simulink model "slrt_ex_pmsm_original_2022b"  (R2022b)
settings: Solver=FixedStepDiscrete  StartTime=0.0  StopTime=0.25  RelTol=1e-3  EnableMultiTasking=on
PreLoadFcn:
  | Ts = 1e-4;
  | Tcpu = 50e-6; %Controller sample time
  | 
  | % PMSM parameters
  | PM = 0.03; % Permanent magnet flux linkage
  | Ld = 2e-4;  % d-axis inductance
  | Lq = 2e-4;  % q-axis inductance
  | L0 = 2e-4;  % 0-axis inductance
  | Rs = 0.013; % Stator resistance
  | N = 6; % Number of pole pairs
  | J = 0.2; % Moment of inertia
  | 
  | % encoder parameters
  | numSlits = 2000; % number of slits
  | pulseSigOffset = 0; % index pulse signal offset
  | shaftInitPos = 0; % motor shaft initial position
  | 
  | % DAC parameters
  | gain = 0.1;
  | bias = 0;
  | 
  | % circuit parameters
  | Vdc = 48;
  | 
  | % real-time parameters
  | ts_FPGA_clk = 5e-9;
  | ts_FPGA_mdl = 1e-6;
  | 
  | % Real-time processor or embedded controller
  | RTorTTL = 1; % 1: Real-time processor,    0: embedded controller
  | 
  | % sample times
  | f_base = 200e6;
  | PWM_frequency = 20e3;
  | ts_FPGA_clk = 1/f_base;
  | ts_FPGA_mdl =1e-6;
libraries: HDL_Motor_Lib x3, hdlsllib x3, SCA_HDL_CoreMath_Lib x1, simulink x1
settings Model: Creator=The MathWorks, Inc.  LastModifiedBy=mathieu.lu-dac
settings OptimizationCC: BlockReduction=off  ConditionallyExecuteInputs=off  DefaultParameterBehavior=Inlined
settings DebuggingCC: AlgebraicLoopMsg=error  SingleTaskRateTransMsg=error  ParameterPrecisionLossMsg=none
settings HardwareCC: ProdBitPerPointer=32  ProdBitPerSizeT=32  ProdBitPerPtrDiffT=32  ProdLargestAtomicFloat=None  ProdIntDivRoundTo=Undefined  ProdEndianess=Unspecified  ProdWordSize=32  ProdHWDeviceType=ASIC/FPGA->ASIC/FPGA  TargetBitPerPointer=64  TargetBitPerSizeT=64  TargetBitPerPtrDiffT=64  TargetLongLongMode=on  TargetIntDivRoundTo=Zero  TargetEndianess=LittleEndian  TargetWordSize=64  TargetHWDeviceType=Custom Processor->MATLAB Host Computer  ProdEqTarget=off
settings ModelReferenceCC: EnableRefExpFcnMdlSchedulingChecks=on
settings RTWCC: DLArmComputeVersion=19.05

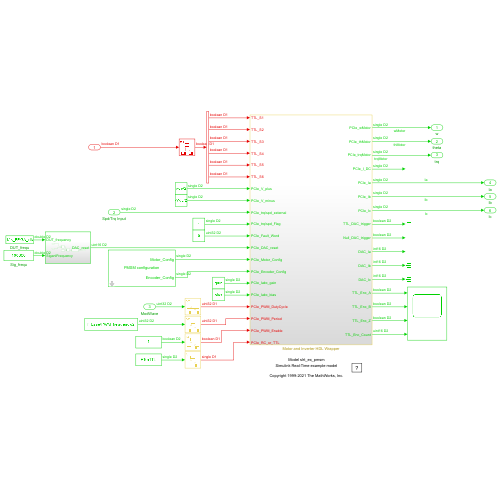
[thumbnail: Simulink's stored preview of the top-level diagram]
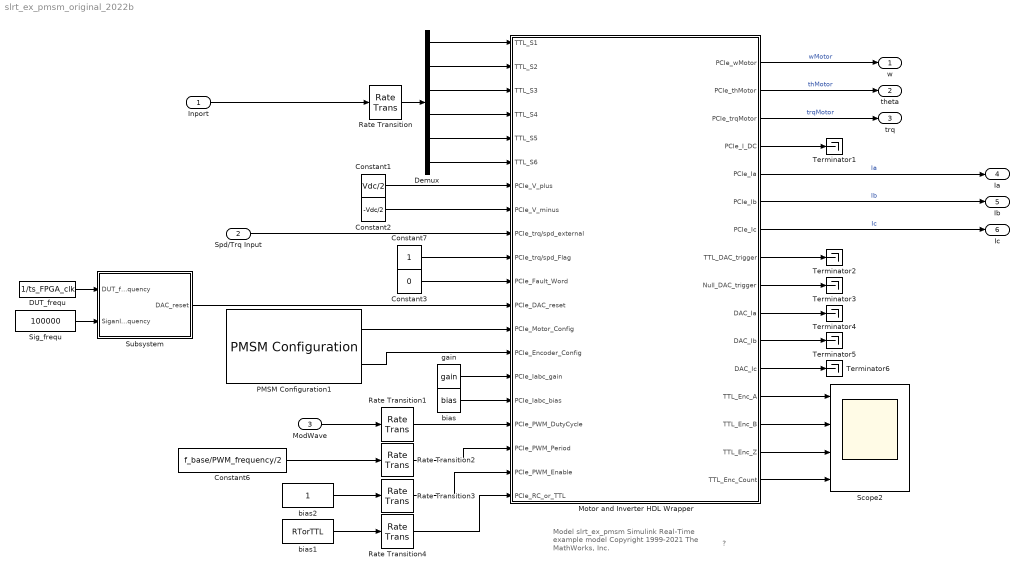
== system slrt_ex_pmsm_original_2022b ==
  note: Model slrt_ex_pmsm
      | Simulink Real-Time example model
      |
      | Copyright 1999-2021 The MathWorks, Inc.
  note: ?
  Inport : Inport  OutDataTypeStr=boolean  PortDimensions=[1 6]
  Spd/Trq Input : Inport  Port=2  OutDataTypeStr=single
  ModWave : Inport  Port=3  OutDataTypeStr=uint32  PortDimensions=[1 3]  SampleTime=ts_FPGA_mdl
  Constant1 : Constant  Value=Vdc/2  OutDataTypeStr=single  SampleTime=ts_FPGA_mdl
  Constant2 : Constant  Value=-Vdc/2  OutDataTypeStr=single  SampleTime=ts_FPGA_mdl
  Constant3 : Constant  Value=0  OutDataTypeStr=uint32  SampleTime=ts_FPGA_mdl
  Constant6 : Constant  Value=f_base/PWM_frequency/2  OutDataTypeStr=uint32  SampleTime=ts_FPGA_mdl
  Constant7 : Constant  OutDataTypeStr=single  SampleTime=ts_FPGA_mdl
  DUT_frequ : Constant  Value=1/ts_FPGA_clk  SampleTime=ts_FPGA_mdl
  Demux : Demux  Outputs=6
  Motor and Inverter HDL Wrapper : Subsystem
  PMSM Configuration1 : HDL_Motor_Lib/PMSM Configuration  Ts=ts_FPGA_mdl  NPP=N  Lambda_pm=PM  Ld=Ld  Lq=Lq  Rs=Rs  J=J  numSlits=numSlits  shaftRotateDir=clockwise (CW)  shaftRotateDirIdx=1  zOffset=pulseSigOffset  shaftInitialPos=shaftInitPos  zGateMode=pulse width = 180 el when channel A is high  zGateModeIdx=1
  Rate Transition{,1..4} (5 alike) : RateTransition  OutPortSampleTime=ts_FPGA_clk
  Scope2 : Scope  NumInputPorts=4
  Sig_frequ : Constant  Value=100000  VectorParams1D=off  SampleTime=ts_FPGA_mdl
  Subsystem : Subsystem
  Terminator{1..6} (6 alike) : Terminator
  bias : Constant  Value=bias  OutDataTypeStr=single  SampleTime=ts_FPGA_mdl
  bias1 : Constant  Value=RTorTTL  OutDataTypeStr=single  SampleTime=ts_FPGA_mdl
  bias2 : Constant  OutDataTypeStr=boolean  SampleTime=ts_FPGA_mdl
  gain : Constant  Value=gain  OutDataTypeStr=single  SampleTime=ts_FPGA_mdl
  w : Outport
  theta : Outport  Port=2
  trq : Outport  Port=3
  Ia : Outport  Port=4
  Ib : Outport  Port=5
  Ic : Outport  Port=6
  wires:
  Rate Transition/1 -> Demux/1
  Demux/1 -> Motor and Inverter HDL Wrapper/1(TTL_S1)
  Demux/2 -> Motor and Inverter HDL Wrapper/2(TTL_S2)
  Demux/3 -> Motor and Inverter HDL Wrapper/3(TTL_S3)
  Demux/4 -> Motor and Inverter HDL Wrapper/4(TTL_S4)
  Demux/5 -> Motor and Inverter HDL Wrapper/5(TTL_S5)
  Demux/6 -> Motor and Inverter HDL Wrapper/6(TTL_S6)
  Constant1/1 -> Motor and Inverter HDL Wrapper/7(PCIe_V_plus)
  Constant2/1 -> Motor and Inverter HDL Wrapper/8(PCIe_V_minus)
  Spd/Trq Input/1 -> Motor and Inverter HDL Wrapper/9(PCIe_trq/spd_external)
  Constant7/1 -> Motor and Inverter HDL Wrapper/10(PCIe_trq/spd_Flag)
  Constant3/1 -> Motor and Inverter HDL Wrapper/11(PCIe_Fault_Word)
  Subsystem/1(DAC_reset) -> Motor and Inverter HDL Wrapper/12(PCIe_DAC_reset)
  Motor and Inverter HDL Wrapper/4(PCIe_I_DC) -> Terminator1/1
  Motor and Inverter HDL Wrapper/8(TTL_DAC_trigger) -> Terminator2/1
  Motor and Inverter HDL Wrapper/9(Null_DAC_trigger) -> Terminator3/1
  Motor and Inverter HDL Wrapper/10(DAC_Ia) -> Terminator4/1
  Motor and Inverter HDL Wrapper/11(DAC_Ib) -> Terminator5/1
  Motor and Inverter HDL Wrapper/12(DAC_Ic) -> Terminator6/1
  Motor and Inverter HDL Wrapper/13(TTL_Enc_A) -> Scope2/1
  Motor and Inverter HDL Wrapper/14(TTL_Enc_B) -> Scope2/2
  Motor and Inverter HDL Wrapper/15(TTL_Enc_Z) -> Scope2/3
  Motor and Inverter HDL Wrapper/16(TTL_Enc_Count) -> Scope2/4
  Inport/1 -> Rate Transition/1
  bias/1 -> Motor and Inverter HDL Wrapper/16(PCIe_Iabc_bias)
  gain/1 -> Motor and Inverter HDL Wrapper/15(PCIe_Iabc_gain)
  Motor and Inverter HDL Wrapper/1(PCIe_wMotor) -> w/1  "wMotor"
  Motor and Inverter HDL Wrapper/2(PCIe_thMotor) -> theta/1  "thMotor"
  Motor and Inverter HDL Wrapper/5(PCIe_Ia) -> Ia/1  "Ia"
  Motor and Inverter HDL Wrapper/6(PCIe_Ib) -> Ib/1  "Ib"
  Motor and Inverter HDL Wrapper/7(PCIe_Ic) -> Ic/1  "Ic"
  DUT_frequ/1 -> Subsystem/1(DUT_frequency)
  Sig_frequ/1 -> Subsystem/2(SiganlFrequency)
  Motor and Inverter HDL Wrapper/3(PCIe_trqMotor) -> trq/1  "trqMotor"
  Constant6/1 -> Rate Transition2/1
  Rate Transition1/1 -> Motor and Inverter HDL Wrapper/17(PCIe_PWM_DutyCycle)
  Rate Transition2/1 -> Motor and Inverter HDL Wrapper/18(PCIe_PWM_Period)
  bias2/1 -> Rate Transition3/1
  Rate Transition3/1 -> Motor and Inverter HDL Wrapper/19(PCIe_PWM_Enable)
  bias1/1 -> Rate Transition4/1
  Rate Transition4/1 -> Motor and Inverter HDL Wrapper/20(PCIe_RC_or_TTL)
  PMSM Configuration1/1 -> Motor and Inverter HDL Wrapper/13(PCIe_Motor_Config)
  PMSM Configuration1/2 -> Motor and Inverter HDL Wrapper/14(PCIe_Encoder_Config)
  ModWave/1 -> Rate Transition1/1

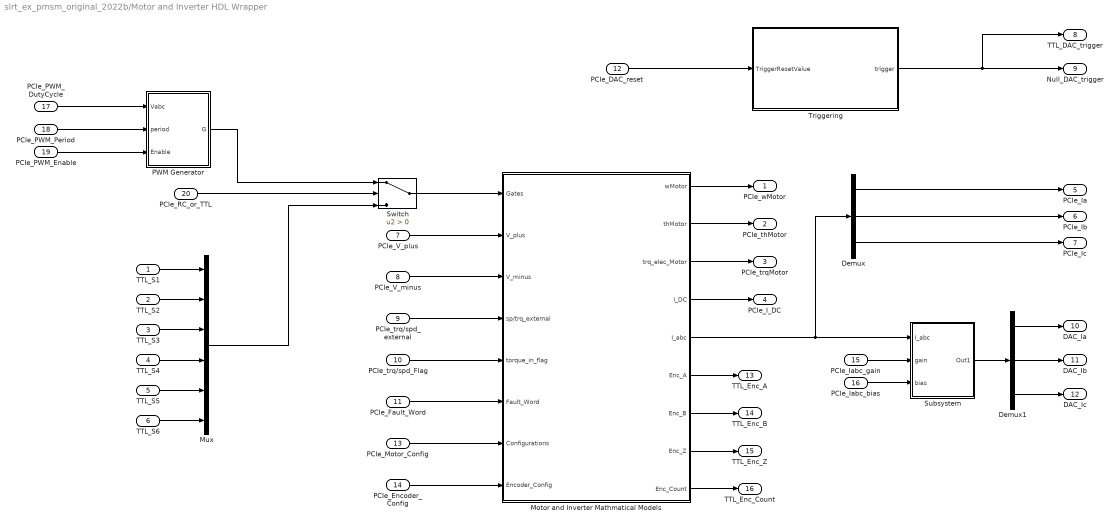
== system slrt_ex_pmsm_original_2022b/Motor and Inverter HDL Wrapper ==
  TTL_S1 : Inport
  TTL_S2 : Inport  Port=2
  TTL_S3 : Inport  Port=3
  TTL_S4 : Inport  Port=4
  TTL_S5 : Inport  Port=5
  TTL_S6 : Inport  Port=6
  PCIe_V_plus : Inport  Port=7
  PCIe_V_minus : Inport  Port=8
  PCIe_trq/spd_external : Inport  Port=9
  PCIe_trq/spd_Flag : Inport  Port=10
  PCIe_Fault_Word : Inport  Port=11
  PCIe_DAC_reset : Inport  Port=12
  PCIe_Motor_Config : Inport  Port=13
  PCIe_Encoder_Config : Inport  Port=14
  PCIe_Iabc_gain : Inport  Port=15
  PCIe_Iabc_bias : Inport  Port=16
  PCIe_PWM_DutyCycle : Inport  Port=17
  PCIe_PWM_Period : Inport  Port=18
  PCIe_PWM_Enable : Inport  Port=19
  PCIe_RC_or_TTL : Inport  Port=20
  Demux : Demux  Outputs=3
  Demux1 : Demux  Outputs=3
  Motor and Inverter Mathmatical Models : Subsystem
  Mux : Mux  Inputs=6
  PWM Generator : Subsystem
  Subsystem : Subsystem
  Switch : Switch  Criteria=u2 > Threshold  SaturateOnIntegerOverflow=off  InputSameDT=off
  Triggering : Subsystem
  PCIe_wMotor : Outport
  PCIe_thMotor : Outport  Port=2
  PCIe_trqMotor : Outport  Port=3
  PCIe_I_DC : Outport  Port=4
  PCIe_Ia : Outport  Port=5
  PCIe_Ib : Outport  Port=6
  PCIe_Ic : Outport  Port=7
  TTL_DAC_trigger : Outport  Port=8
  Null_DAC_trigger : Outport  Port=9
  DAC_Ia : Outport  Port=10
  DAC_Ib : Outport  Port=11
  DAC_Ic : Outport  Port=12
  TTL_Enc_A : Outport  Port=13
  TTL_Enc_B : Outport  Port=14
  TTL_Enc_Z : Outport  Port=15
  TTL_Enc_Count : Outport  Port=16
  wires:
  Motor and Inverter Mathmatical Models/3(trq_elec_Motor) -> PCIe_trqMotor/1
  Motor and Inverter Mathmatical Models/2(thMotor) -> PCIe_thMotor/1
  Triggering/1(trigger) -> Null_DAC_trigger/1, TTL_DAC_trigger/1
  Demux/2 -> PCIe_Ib/1
  Motor and Inverter Mathmatical Models/1(wMotor) -> PCIe_wMotor/1
  Demux/1 -> PCIe_Ia/1
  TTL_S2/1 -> Mux/2
  Motor and Inverter Mathmatical Models/4(I_DC) -> PCIe_I_DC/1
  PCIe_trq/spd_external/1 -> Motor and Inverter Mathmatical Models/4(sp/trq_external)
  Demux/3 -> PCIe_Ic/1
  PCIe_V_plus/1 -> Motor and Inverter Mathmatical Models/2(V_plus)
  PCIe_trq/spd_Flag/1 -> Motor and Inverter Mathmatical Models/5(torque_in_flag)
  TTL_S3/1 -> Mux/3
  PCIe_V_minus/1 -> Motor and Inverter Mathmatical Models/3(V_minus)
  TTL_S6/1 -> Mux/6
  TTL_S1/1 -> Mux/1
  TTL_S5/1 -> Mux/5
  PCIe_Encoder_Config/1 -> Motor and Inverter Mathmatical Models/8(Encoder_Config)
  TTL_S4/1 -> Mux/4
  Motor and Inverter Mathmatical Models/6(Enc_A) -> TTL_Enc_A/1
  PCIe_Fault_Word/1 -> Motor and Inverter Mathmatical Models/6(Fault_Word)
  Motor and Inverter Mathmatical Models/5(I_abc) -> Demux/1, Subsystem/1(I_abc)
  PCIe_DAC_reset/1 -> Triggering/1(TriggerResetValue)
  PCIe_Motor_Config/1 -> Motor and Inverter Mathmatical Models/7(Configurations)
  Motor and Inverter Mathmatical Models/9(Enc_Count) -> TTL_Enc_Count/1
  Motor and Inverter Mathmatical Models/7(Enc_B) -> TTL_Enc_B/1
  Motor and Inverter Mathmatical Models/8(Enc_Z) -> TTL_Enc_Z/1
  PCIe_Iabc_gain/1 -> Subsystem/2(gain)
  PCIe_Iabc_bias/1 -> Subsystem/3(bias)
  Subsystem/1(Out1) -> Demux1/1
  Demux1/2 -> DAC_Ib/1
  Demux1/1 -> DAC_Ia/1
  Demux1/3 -> DAC_Ic/1
  PCIe_PWM_DutyCycle/1 -> PWM Generator/1(Vabc)
  PCIe_PWM_Period/1 -> PWM Generator/2(period)
  PCIe_PWM_Enable/1 -> PWM Generator/3(Enable)
  PWM Generator/1(G) -> Switch/1
  Switch/1 -> Motor and Inverter Mathmatical Models/1(Gates)
  Mux/1 -> Switch/3
  PCIe_RC_or_TTL/1 -> Switch/2

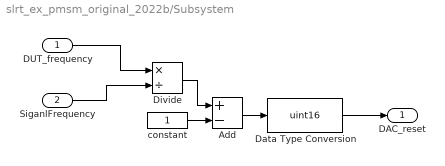
== system slrt_ex_pmsm_original_2022b/Subsystem ==
  DUT_frequency : Inport
  SiganlFrequency : Inport  Port=2
  Add : Sum  Inputs=+-
  Data Type Conversion : DataTypeConversion  OutDataTypeStr=uint16  SaturateOnIntegerOverflow=off  RndMeth=Floor
  Divide : Product  Inputs=*/
  constant : Constant  VectorParams1D=off  SampleTime=-1
  DAC_reset : Outport
  wires:
  DUT_frequency/1 -> Divide/1
  constant/1 -> Add/2
  Data Type Conversion/1 -> DAC_reset/1
  Divide/1 -> Add/1
  Add/1 -> Data Type Conversion/1
  SiganlFrequency/1 -> Divide/2

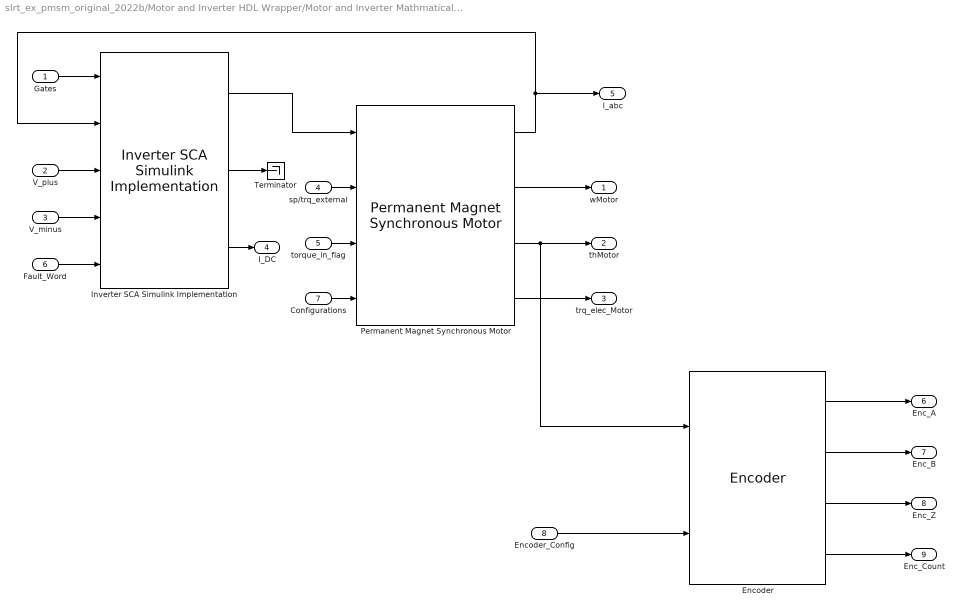
== system slrt_ex_pmsm_original_2022b/Motor and Inverter HDL Wrapper/Motor and Inverter Mathmatical Models ==
  Gates : Inport
  V_plus : Inport  Port=2
  V_minus : Inport  Port=3
  sp/trq_external : Inport  Port=4
  torque_in_flag : Inport  Port=5
  Fault_Word : Inport  Port=6
  Configurations : Inport  Port=7
  Encoder_Config : Inport  Port=8
  Encoder : HDL_Motor_Lib/Encoder
  Inverter SCA Simulink Implementation : SCA_HDL_CoreMath_Lib/Inverter SCA Simulink Implementation  rSwitch=0.001  vfSwitch=0.1  rDiode=0.001  vfDiode=0.8  rSnub=100  ts_Model=ts_FPGA_mdl  ts_FPGA=ts_FPGA_clk
  Permanent Magnet Synchronous Motor : HDL_Motor_Lib/Permanent Magnet Synchronous Motor  Ts=ts_FPGA_mdl
  Terminator : Terminator
  wMotor : Outport
  thMotor : Outport  Port=2
  trq_elec_Motor : Outport  Port=3
  I_DC : Outport  Port=4
  I_abc : Outport  Port=5
  Enc_A : Outport  Port=6
  Enc_B : Outport  Port=7
  Enc_Z : Outport  Port=8
  Enc_Count : Outport  Port=9
  wires:
  torque_in_flag/1 -> Permanent Magnet Synchronous Motor/3
  Permanent Magnet Synchronous Motor/4 -> trq_elec_Motor/1
  Permanent Magnet Synchronous Motor/3 -> thMotor/1, Encoder/1
  Inverter SCA Simulink Implementation/2 -> Terminator/1
  V_plus/1 -> Inverter SCA Simulink Implementation/3
  Gates/1 -> Inverter SCA Simulink Implementation/1
  Configurations/1 -> Permanent Magnet Synchronous Motor/4
  Encoder/4 -> Enc_Count/1
  Encoder/2 -> Enc_B/1
  Encoder/3 -> Enc_Z/1
  Encoder/1 -> Enc_A/1
  Permanent Magnet Synchronous Motor/1 -> I_abc/1, Inverter SCA Simulink Implementation/2
  Inverter SCA Simulink Implementation/1 -> Permanent Magnet Synchronous Motor/1
  sp/trq_external/1 -> Permanent Magnet Synchronous Motor/2
  Permanent Magnet Synchronous Motor/2 -> wMotor/1
  Fault_Word/1 -> Inverter SCA Simulink Implementation/5
  Inverter SCA Simulink Implementation/3 -> I_DC/1
  V_minus/1 -> Inverter SCA Simulink Implementation/4
  Encoder_Config/1 -> Encoder/2

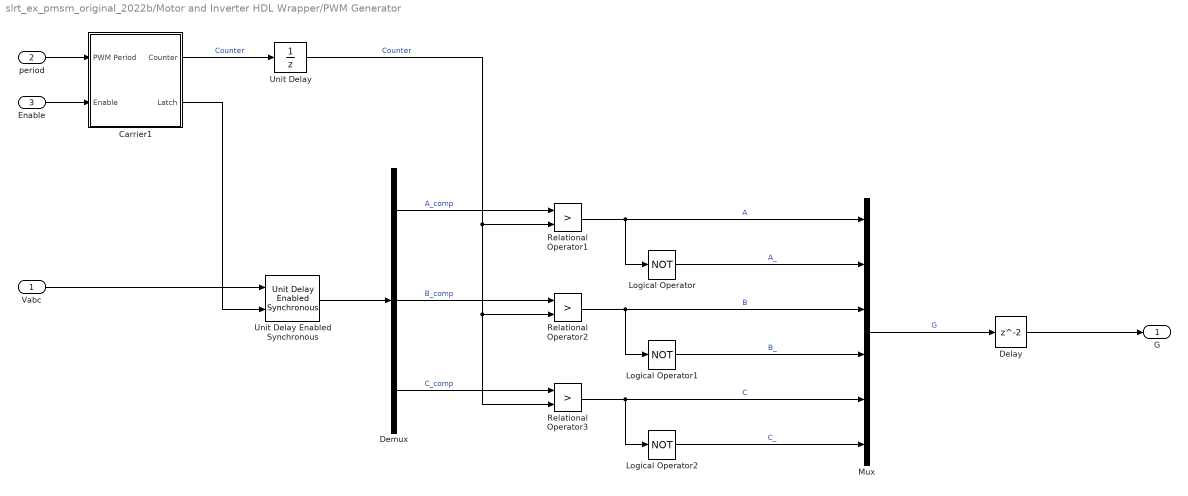
== system slrt_ex_pmsm_original_2022b/Motor and Inverter HDL Wrapper/PWM Generator ==
  Vabc : Inport
  period : Inport  Port=2
  Enable : Inport  Port=3
  Carrier1 : Subsystem
  Delay : Delay
  Demux : Demux  Outputs=3
  Logical Operator : Logic  Operator=NOT  AllPortsSameDT=off  OutDataTypeStr=boolean
  Logical Operator1 : Logic  Operator=NOT  AllPortsSameDT=off  OutDataTypeStr=boolean
  Logical Operator2 : Logic  Operator=NOT  AllPortsSameDT=off  OutDataTypeStr=boolean
  Mux : Mux  Inputs=6
  Relational Operator1 : RelationalOperator  Operator=>  OutDataTypeStr=boolean  InputSameDT=off
  Relational Operator2 : RelationalOperator  Operator=>  OutDataTypeStr=boolean  InputSameDT=off
  Relational Operator3 : RelationalOperator  Operator=>  OutDataTypeStr=boolean  InputSameDT=off
  Unit Delay : UnitDelay  SampleTime=-1  HasFrameUpgradeWarning=on
  Unit Delay Enabled Synchronous : hdlsllib/Discrete/Unit Delay Enabled Synchronous  InitialCondition=0.0  SampleTime=-1
  G : Outport  VectorParamsAs1DForOutWhenUnconnected=off
  wires:
  period/1 -> Carrier1/1(PWM Period)
  Demux/2 -> Relational Operator2/1  "B_comp"
  Logical Operator2/1 -> Mux/6  "C_"
  Relational Operator3/1 -> Mux/5, Logical Operator2/1  "C"
  Logical Operator/1 -> Mux/2  "A_"
  Vabc/1 -> Unit Delay Enabled Synchronous/1
  Logical Operator1/1 -> Mux/4  "B_"
  Unit Delay/1 -> Relational Operator1/2, Relational Operator3/2, Relational Operator2/2  "Counter"
  Demux/1 -> Relational Operator1/1  "A_comp"
  Demux/3 -> Relational Operator3/1  "C_comp"
  Relational Operator1/1 -> Logical Operator/1, Mux/1  "A"
  Relational Operator2/1 -> Mux/3, Logical Operator1/1  "B"
  Carrier1/2(Latch) -> Unit Delay Enabled Synchronous/2
  Unit Delay Enabled Synchronous/1 -> Demux/1
  Carrier1/1(Counter) -> Unit Delay/1  "Counter"
  Enable/1 -> Carrier1/2(Enable)
  Mux/1 -> Delay/1  "G"
  Delay/1 -> G/1

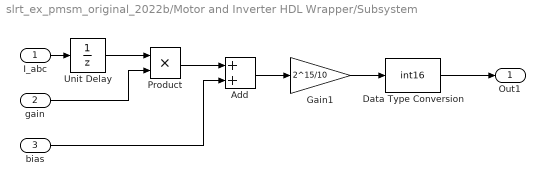
== system slrt_ex_pmsm_original_2022b/Motor and Inverter HDL Wrapper/Subsystem ==
  I_abc : Inport
  gain : Inport  Port=2
  bias : Inport  Port=3
  Add : Sum
  Data Type Conversion : DataTypeConversion  OutDataTypeStr=int16  RndMeth=Nearest  SaturateOnIntegerOverflow=off
  Gain1 : Gain  Gain=2^15/10
  Product : Product
  Unit Delay : UnitDelay  SampleTime=-1  HasFrameUpgradeWarning=on
  Out1 : Outport
  wires:
  Product/1 -> Add/1
  Unit Delay/1 -> Product/1
  Data Type Conversion/1 -> Out1/1
  Add/1 -> Gain1/1
  bias/1 -> Add/2
  I_abc/1 -> Unit Delay/1
  Gain1/1 -> Data Type Conversion/1
  gain/1 -> Product/2

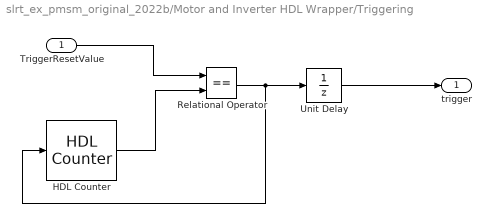
== system slrt_ex_pmsm_original_2022b/Motor and Inverter HDL Wrapper/Triggering ==
  TriggerResetValue : Inport
  HDL Counter : hdlsllib/Sources/HDL Counter  CountType=Free running  CountInit=0  CountStep=1  CountMax=25  CountFromType=Initial value  CountFrom=0  CountResetPort=on  CountLoadPort=off  CountEnbPort=off  CountDirPort=off  CountHitOutputPort=off  CountDataType=Unsigned  CountWordLen=16  CountFracLen=0  CountSampTime=1
  Relational Operator : RelationalOperator  Operator===  OutDataTypeStr=boolean  InputSameDT=off
  Unit Delay : UnitDelay  SampleTime=-1  HasFrameUpgradeWarning=on
  trigger : Outport
  wires:
  TriggerResetValue/1 -> Relational Operator/1
  HDL Counter/1 -> Relational Operator/2
  Relational Operator/1 -> HDL Counter/1, Unit Delay/1
  Unit Delay/1 -> trigger/1

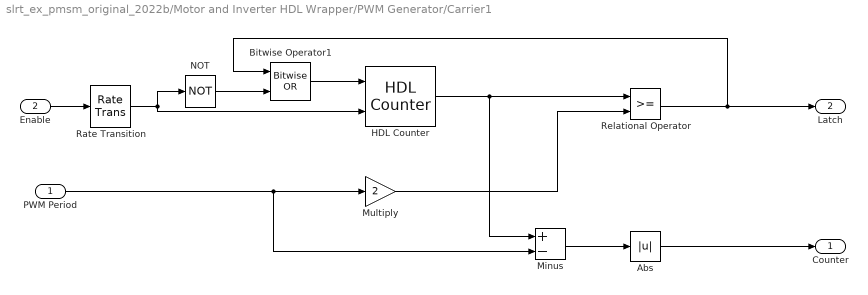
== system slrt_ex_pmsm_original_2022b/Motor and Inverter HDL Wrapper/PWM Generator/Carrier1 ==
  PWM Period : Inport  OutDataTypeStr=uint32  PortDimensions=1
  Enable : Inport  Port=2  OutDataTypeStr=boolean  PortDimensions=1
  Abs : Abs  OutDataTypeStr=uint32  SaturateOnIntegerOverflow=off
  Bitwise Operator1 : simulink/Logic and Bit Operations/Bitwise Operator  logicop=OR  UseBitMask=off  NumInputPorts=2  BitMask=bin2dec('11011001')  BitMaskRealWorld=Stored Integer
  HDL Counter : hdlsllib/Sources/HDL Counter  CountType=Free running  CountInit=0  CountStep=1  CountMax=25  CountFromType=Initial value  CountFrom=0  CountResetPort=on  CountLoadPort=off  CountEnbPort=on  CountDirPort=off  CountHitOutputPort=off  CountDataType=Unsigned  CountWordLen=32  CountFracLen=0  CountSampTime=1
  Minus : Sum  Inputs=+-  OutDataTypeStr=int32
  Multiply : Gain  Gain=2  OutDataTypeStr=uint32
  NOT : Logic  Operator=NOT  AllPortsSameDT=off  OutDataTypeStr=boolean
  Rate Transition : RateTransition
  Relational Operator : RelationalOperator  OutDataTypeStr=boolean  InputSameDT=off
  Counter : Outport  VectorParamsAs1DForOutWhenUnconnected=off
  Latch : Outport  Port=2
  wires:
  Rate Transition/1 -> NOT/1, HDL Counter/2
  HDL Counter/1 -> Relational Operator/1, Minus/1
  PWM Period/1 -> Multiply/1, Minus/2
  Minus/1 -> Abs/1
  Abs/1 -> Counter/1
  Multiply/1 -> Relational Operator/2
  Relational Operator/1 -> Bitwise Operator1/1, Latch/1
  NOT/1 -> Bitwise Operator1/2
  Bitwise Operator1/1 -> HDL Counter/1
  Enable/1 -> Rate Transition/1
